simulink model "part3_batterychargingchanged"  (R2022b)
settings: Solver=VariableStepAuto  StartTime=0.0  StopTime=120  RelTol=1e-3
undefined symbols (not defined in the file): High, Low
libraries: fl_lib x6, nesl_utility x6, ee_lib x3, batteryecm_lib x1
settings Model: Creator=mingreico  LastModifiedBy=mingreico

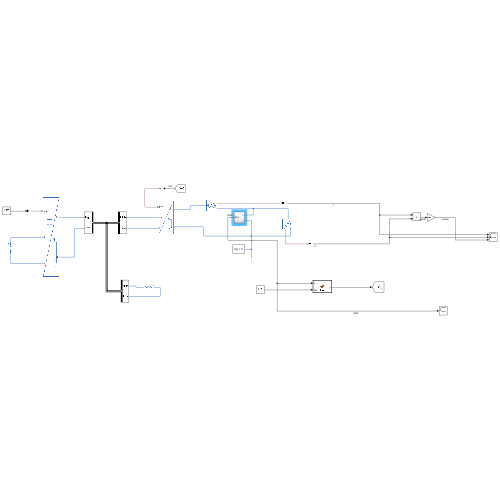
[thumbnail: Simulink's stored preview of the top-level diagram]
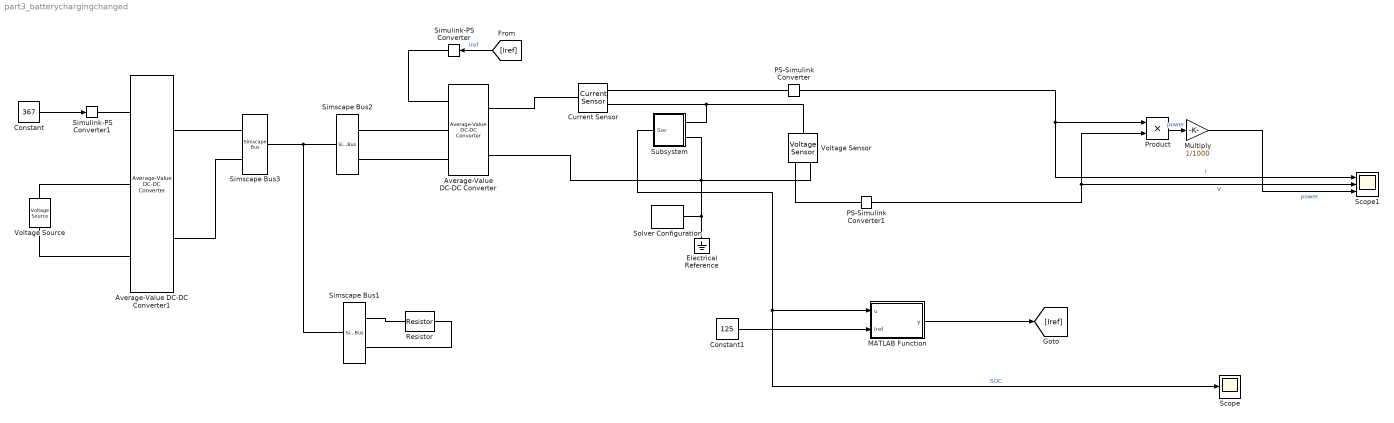
== system part3_batterychargingchanged ==
  Average-Value DC-DC Converter : ee_lib/Semiconductors & Converters/Converters/Average-Value DC-DC Converter  control_option=ee.enum.converters.controlinput.current  converter_type=ee.enum.converters.dcdctype.buckboost  efficiency_option=ee.enum.converters.efficiency.constant  efficiency_fixed=100  i_vec=[0, 2, 5] A  efficiency_vec=[90, 95, 98]
      settings: InternalSimscapePortConfiguration="{\"Bottom\":[],\"Left\":[{\"id\":\"Iref\",\"label\":\"Iref\",\"type\":\"input\"},{\"id\":\"p1\",\"label\":\"1+\",\"type\":\"foundation.electrical.electrical\"},{\"id\":\"n1\",\"label\":\"1-\",\"type\":\"foundation.electrical.electrical\"}],\"Right\":[{\"id\":\"p2\",\"label\":\"2+\",\"type\":\"foundation.electrical.electrical\"},{\"id\":\"n2\",\"label\":\"2-\",\"type\":\"foundation.electrical.electrical\"}],\"Top\":[]}"
  Average-Value DC-DC Converter1 : ee_lib/Semiconductors & Converters/Converters/Average-Value DC-DC Converter  control_option=ee.enum.converters.controlinput.voltage  converter_type=ee.enum.converters.dcdctype.buck  efficiency_option=ee.enum.converters.efficiency.constant  efficiency_fixed=100  i_vec=[0, 2, 5] A  efficiency_vec=[90, 95, 98]
      settings: InternalSimscapePortConfiguration="{\"Bottom\":[],\"Left\":[{\"id\":\"Vref\",\"label\":\"Vref\",\"type\":\"input\"},{\"id\":\"p1\",\"label\":\"1+\",\"type\":\"foundation.electrical.electrical\"},{\"id\":\"n1\",\"label\":\"1-\",\"type\":\"foundation.electrical.electrical\"}],\"Right\":[{\"id\":\"p2\",\"label\":\"2+\",\"type\":\"foundation.electrical.electrical\"},{\"id\":\"n2\",\"label\":\"2-\",\"type\":\"foundation.electrical.electrical\"}],\"Top\":[]}"
  Constant : Constant  Value=367
  Constant1 : Constant  Value=125
  Current Sensor : fl_lib/Electrical/Electrical Sensors/Current Sensor
  Electrical Reference : fl_lib/Electrical/Electrical Elements/Electrical Reference
  MATLAB Function : MATLAB Function  TreatAsAtomicUnit=on
  Multiply : Gain  Gain=1/1000
  PS-Simulink Converter : nesl_utility/PS-Simulink Converter  PhysicalDomain=network_engine_domain  SubClassName=ps_output  LeftPortType=input  RightPortType=output  PseudoPeriodic=off  Frequencies=[]  VectorFormat=inherit  Unit=inherit  AffineConversion=off
  PS-Simulink Converter1 : nesl_utility/PS-Simulink Converter  PhysicalDomain=network_engine_domain  SubClassName=ps_output  LeftPortType=input  RightPortType=output  PseudoPeriodic=off  Frequencies=[]  VectorFormat=inherit  Unit=inherit  AffineConversion=off
  Product : Product
  Resistor : fl_lib/Electrical/Electrical Elements/Resistor  R=1000 Ohm  i_specify=off  i_priority=None  i=0 A  i_nominal_specify=off  i_nominal_unit=A  i_nominal_value=1  v_specify=off  v_priority=None  v=0 V  v_nominal_specify=off  v_nominal_unit=V  v_nominal_value=1
  Scope : Scope
  Scope1 : Scope  NumInputPorts=3
  Simscape Bus1 : SimscapeBus  HierarchyStrings=High;Low
  Simscape Bus2 : SimscapeBus  HierarchyStrings=High;Low
  Simscape Bus3 : SimscapeBus  HierarchyStrings=High;Low
  Simulink-PS Converter : nesl_utility/Simulink-PS Converter  PhysicalDomain=network_engine_domain  SubClassName=ps_input  LeftPortType=input  RightPortType=output  PseudoPeriodic=off  Frequencies=[]  NoiseDistribution=none  NoiseParameters=[]  Unit=1  AffineConversion=off  FilteringAndDerivatives=provide  SimscapeFilterOrder=1  InputFilterTimeConstant=0.001  UdotUserProvided=0
  Simulink-PS Converter1 : nesl_utility/Simulink-PS Converter  PhysicalDomain=network_engine_domain  SubClassName=ps_input  LeftPortType=input  RightPortType=output  PseudoPeriodic=off  Frequencies=[]  NoiseDistribution=none  NoiseParameters=[]  Unit=1  AffineConversion=off  FilteringAndDerivatives=provide  SimscapeFilterOrder=1  InputFilterTimeConstant=0.001  UdotUserProvided=0
  Solver Configuration : nesl_utility/Solver Configuration  PhysicalDomain=network_engine_domain  SubClassName=solver  LeftPortType=input  RightPortType=generic  Tones=[]  Harmonics=[]  SimulateNoise=off  Profile=off  UseLocalSampling=off  EnableSwitchedLinearOptims=on  FrequencyDomain=off  UseCCode=off  RelTol=0.001  AbsTol=0.001  MinStep=1e-09  ToWorkspace=off  RevertToSquareIcSolve=off  NumHomotopyIterations=100  PhasorMode=off  PhasorModeNumHarmonics=1  ConsistencySolver=NEWTON_XTOL_AFTER_FTOL  IndexReductionMethod=DerivativeReplacement  DoDC=off  ResidualTolerance=1e-09  ConsistencyTolSource=GLOBAL  ConsistencyAbsTol=0.001  ConsistencyRelTol=0.001  ConsistencyTolFactor=0.001  UseLocalSolver=off  LocalSolverChoice=NE_BACKWARD_EULER_ADVANCER  ResolveIndetEquations=on  FunctionEvalNumThread=1  LocalSolverSampleTime=0.001  DoFixedCost=off  MaxNonlinIter=3  MaxModeIter=2  ComputeImpulses=off  ImpulseIterations=2  LinearAlgebra=auto  LinearAlgebraNumThread=0  EquationFormulation=NE_TIME_EF  DelaysMemoryBudget=1024  AutomaticFiltering=on  FilteringTimeConstant=0.001  PartitionStorageMethod=AS_NEEDED  PartitionMemoryBudget=1024  PartitionMethod=ROBUST
  Subsystem : Subsystem
  Voltage Sensor : fl_lib/Electrical/Electrical Sensors/Voltage Sensor
  Voltage Source : ee_lib/Sources/Voltage Source  dc_voltage=1000 V  ac_voltage=0 V  ac_shift=0 rad  ac_frequency=60 Hz  noise_mode=ee.enum.sources.noise.Disabled  PSD=0 V^2/Hz  sample_time=1e-3 s  repeatability=ee.enum.sources.repeatability.NotRepeatable  user_seed=0  auto_seed=3890346746  i_specify=off  i_priority=None  i=0 A  i_nominal_specify=off  i_nominal_unit=A  i_nominal_value=1  v_specify=off  v_priority=None  v=0 V  v_nominal_specify=off  v_nominal_unit=V  v_nominal_value=1
  wires:
  PS-Simulink Converter/1 -> Scope1/1, Product/1  "I"
  PS-Simulink Converter1/1 -> Product/2, Scope1/2  "V"
  [Iref] -> Simulink-PS Converter/1  "iref"
  MATLAB Function/1(y) -> [Iref]
  Constant/1 -> Simulink-PS Converter1/1
  Subsystem/1(Soc) -> Scope/1, MATLAB Function/1(u)  "SOC"
  Constant1/1 -> MATLAB Function/2(Iref)
  Product/1 -> Multiply/1  "power"
  Multiply/1 -> Scope1/3  "power"
  connections:
  Current Sensor/RConn2 -- Voltage Sensor/LConn1 -- Subsystem/LConn1
  Current Sensor/RConn1 -- PS-Simulink Converter/LConn1
  Voltage Sensor/RConn1 -- PS-Simulink Converter1/LConn1
  Simulink-PS Converter/RConn1 -- Average-Value DC-DC Converter/LConn1
  Voltage Source/RConn1 -- Average-Value DC-DC Converter1/LConn3
  Simulink-PS Converter1/RConn1 -- Average-Value DC-DC Converter1/LConn1
  Voltage Source/LConn1 -- Average-Value DC-DC Converter1/LConn2
  Simscape Bus3/LConn1 -- Average-Value DC-DC Converter1/RConn1
  Average-Value DC-DC Converter1/RConn2 -- Simscape Bus3/LConn2
  Simscape Bus2/RConn1 -- Simscape Bus1/RConn1 -- Simscape Bus3/RConn1
  Average-Value DC-DC Converter/LConn2 -- Simscape Bus2/LConn1
  Simscape Bus2/LConn2 -- Average-Value DC-DC Converter/LConn3
  Subsystem/LConn2 -- Voltage Sensor/RConn2 -- Average-Value DC-DC Converter/RConn2 -- Solver Configuration/RConn1 -- Electrical Reference/LConn1
  Current Sensor/LConn1 -- Average-Value DC-DC Converter/RConn1
  Resistor/LConn1 -- Simscape Bus1/LConn1
  Resistor/RConn1 -- Simscape Bus1/LConn2

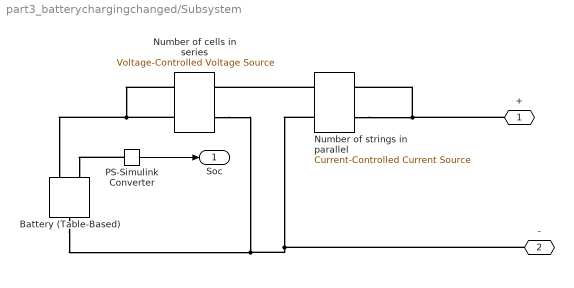
== system part3_batterychargingchanged/Subsystem ==
  Battery (Table-Based) : batteryecm_lib/Battery (Table-Based)  Tag={'toolbox/physmod/battery/shared_library/m/batteryecm_lib_parts';'Battery__Table_Based_/Panasonic/NCR18650PF.xml'}  SOC_vec=[0 0.01 0.02 0.03 0.04 0.05 0.06 0.07 0.08 0.09 0.1 0.11 0.12 0.13 0.14 0.15 0.16 0.17 0.18 0.19 0.2 0.21 0.22 0.23 0.24 0.25 0.26 0.27 0.28 0.29 0.3 0.31 0.32 0.33 0.34 0.35 0.36 0.37 0.38 0.39 0.4 0.41 0.42 0.43 0.44 0.45 0.46 0.47 0.48 0.49 0.5 0.51 0.52 0.53 0.54 0.55 0.56 0.57 0.58 0.59 0.6 0.61 0.62 0.63 0.64 0.65 0.66 0.67 0.68 0.69 0.7 0.71 0.72 0.73 0.74 0.75 0.76 0.77 0.78 0.79 0.8 0.81 0.82 0.83 0.84 0.85 0.86 0.87 0.88 0.89 0.9 0.91 0.92 0.93 0.94 0.95 0.96 0.97 0.98 0.99 1]  T_dependence=simscape.enum.tablebattery.temperature_dependence.yes  prm_dir=simscape.enum.tablebattery.prm_dir.noCurrentDirectionality  T_vec=[-10 0 25 45] degC  V0_mat=[2.80555 2.80555 2.80555 2.80555;2.85959 2.85959 2.85959 2.85959;2.91363 2.91363 2.91363 2.91363;3.00304 3.00304 3.00304 3.00304;3.0606 3.0606 3.0606 3.0606;3.09933 3.09933 3.09933 3.09933;3.12978 3.12978 3.12978 3.12978;3.18381 3.18381 3.18381 3.18381;3.23096 3.23096 3.23096 3.23096;3.26469 3.26469 3.26469 3.26469;3.2911 3.2911 3.2911 3.2911;3.31202 3.31202 3.31202 3.31202;3.33368 3.33368 3.33368 3.33368;3.35023 3.35023 3.35023 3.35023;3.3665 3.3665 3.3665 3.3665;3.38187 3.38187 3.38187 3.38187;3.39652 3.39652 3.39652 3.39652;3.40935 3.40935 3.40935 3.40935;3.42296 3.42296 3.42296 3.42296;3.43602 3.43602 3.43602 3.43602;3.4475 3.4475 3.4475 3.4475;3.45894 3.45894 3.45894 3.45894;3.46943 3.46943 3.46943 3.46943;3.47583 3.47583 3.47583 3.47583;3.48131 3.48131 3.48131 3.48131;3.48929 3.48929 3.48929 3.48929;3.49863 3.49863 3.49863 3.49863;3.50723 3.50723 3.50723 3.50723;3.51419 3.51419 3.51419 3.51419;3.52064 3.52064 3.52064 3.52064;3.52703 3.52703 3.52703 3.52703;3.53288 3.53288 3.53288 3.53288;3.5383 3.5383 3.5383 3.5383;3.54248 3.54248 3.54248 3.54248;3.54635 3.54635 3.54635 3.54635;3.55067 3.55067 3.55067 3.55067;3.55538 3.55538 3.55538 3.55538;3.56162 3.56162 3.56162 3.56162;3.56772 3.56772 3.56772 3.56772;3.57355 3.57355 3.57355 3.57355;3.57907 3.57907 3.57907 3.57907;3.58466 3.58466 3.58466 3.58466;3.59099 3.59099 3.59099 3.59099;3.59795 3.59795 3.59795 3.59795;3.60491 3.60491 3.60491 3.60491;3.61176 3.61176 3.61176 3.61176;3.61856 3.61856 3.61856 3.61856;3.62438 3.62438 3.62438 3.62438;3.62996 3.62996 3.62996 3.62996;3.63625 3.63625 3.63625 3.63625;3.64309 3.64309 3.64309 3.64309;3.64978 3.64978 3.64978 3.64978;3.65633 3.65633 3.65633 3.65633;3.66344 3.66344 3.66344 3.66344;3.67149 3.67149 3.67149 3.67149;3.67995 3.67995 3.67995 3.67995;3.68883 3.68883 3.68883 3.68883;3.69977 3.69977 3.69977 3.69977;3.7106 3.7106 3.7106 3.7106;3.72128 3.72128 3.72128 3.72128;3.72977 3.72977 3.72977 3.72977;3.73862 3.73862 3.73862 3.73862;3.74839 3.74839 3.74839 3.74839;3.75854 3.75854 3.75854 3.75854;3.76808 3.76808 3.76808 3.76808;3.77731 3.77731 3.77731 3.77731;3.78691 3.78691 3.78691 3.78691;3.79724 3.79724 3.79724 3.79724;3.80748 3.80748 3.80748 3.80748;3.817 3.817 3.817 3.817;3.82465 3.82465 3.82465 3.82465;3.83227 3.83227 3.83227 3.83227;3.8402 3.8402 3.8402 3.8402;3.84937 3.84937 3.84937 3.84937;3.85948 3.85948 3.85948 3.85948;3.87001 3.87001 3.87001 3.87001;3.88001 3.88001 3.88001 3.88001;3.88909 3.88909 3.88909 3.88909;3.89708 3.89708 3.89708 3.89708;3.90554 3.90554 3.90554 3.90554;3.91623 3.91623 3.91623 3.91623;3.9276 3.9276 3.9276 3.9276;3.9408 3.9408 3.9408 3.9408;3.95458 3.95458 3.95458 3.95458;3.96671 3.96671 3.96671 3.96671;3.97597 3.97597 3.97597 3.97597;3.98588 3.98588 3.98588 3.98588;3.99921 3.99921 3.99921 3.99921;4.01279 4.01279 4.01279 4.01279;4.02654 4.02654 4.02654 4.02654;4.03959 4.03959 4.03959 4.03959;4.05214 4.05214 4.05214 4.05214;4.06294 4.06294 4.06294 4.06294;4.07257 4.07257 4.07257 4.07257;4.08033 4.08033 4.08033 4.08033;4.08863 4.08863 4.08863 4.08863;4.09953 4.09953 4.09953 4.09953;4.11328 4.11328 4.11328 4.11328;4.13091 4.13091 4.13091 4.13091;4.15201 4.15201 4.15201 4.15201;4.17387 4.17387 4.17387 4.17387] V  V0_vec=[2.80555 2.85959 2.91363 3.00304 3.0606 3.09933 3.12978 3.18381 3.23096 3.26469 3.2911 3.31202 3.33368 3.35023 3.3665 3.38187 3.39652 3.40935 3.42296 3.43602 3.4475 3.45894 3.46943 3.47583 3.48131 3.48929 3.49863 3.50723 3.51419 3.52064 3.52703 3.53288 3.5383 3.54248 3.54635 3.55067 3.55538 3.56162 3.56772 3.57355 3.57907 3.58466 3.59099 3.59795 3.60491 3.61176 3.61856 3.62438 3.62996 3.63625 3.64309 3.64978 3.65633 3.66344 3.67149 3.67995 3.68883 3.69977 3.7106 3.72128 3.72977 3.73862 3.74839 3.75854 3.76808 3.77731 3.78691 3.79724 3.80748 3.817 3.82465 3.83227 3.8402 3.84937 3.85948 3.87001 3.88001 3.88909 3.89708 3.90554 3.91623 3.9276 3.9408 3.95458 3.96671 3.97597 3.98588 3.99921 4.01279 4.02654 4.03959 4.05214 4.06294 4.07257 4.08033 4.08863 4.09953 4.11328 4.13091 4.15201 4.17387] V  V_range=[2.25 Inf] V  R0_mat=[0.75549 0.67245 0.17403 0.112;0.85269 0.75703 0.14702 0.03414;0.81792 0.71964 0.12022 0.00255;0.78315 0.68225 0.10415 2e-05;0.74837 0.64486 0.08835 2e-05;0.7136 0.60747 0.07462 2e-05;0.67883 0.57008 0.06392 2e-05;0.64406 0.53269 0.06243 0.01154;0.60929 0.49529 0.06276 0.02196;0.57452 0.4579 0.06157 0.02895;0.53975 0.42051 0.06015 0.03291;0.50498 0.38312 0.0587 0.03446;0.47021 0.34573 0.05791 0.03749;0.43544 0.30834 0.05742 0.03912;0.40067 0.27163 0.05726 0.04077;0.3659 0.2399 0.05695 0.04312;0.33113 0.21598 0.05669 0.04519;0.29855 0.19556 0.0563 0.04597;0.27187 0.18199 0.05643 0.04689;0.25149 0.16998 0.05637 0.04778;0.23672 0.15947 0.05613 0.04881;0.22094 0.15288 0.05627 0.04983;0.21055 0.14641 0.0562 0.05042;0.19955 0.13998 0.0555 0.04905;0.19137 0.13379 0.05463 0.04734;0.18464 0.13036 0.05424 0.0468;0.17901 0.12743 0.05396 0.04733;0.17336 0.12471 0.05353 0.04759;0.16963 0.12142 0.05325 0.04697;0.16579 0.11998 0.053 0.04616;0.16242 0.11856 0.05273 0.04563;0.15887 0.11696 0.05239 0.04515;0.15558 0.1153 0.05185 0.04523;0.15182 0.11319 0.05104 0.04515;0.14868 0.11098 0.05016 0.04495;0.14619 0.10898 0.0496 0.04427;0.1438 0.10712 0.04917 0.0435;0.14196 0.10583 0.049 0.0433;0.14006 0.10467 0.04873 0.04342;0.13885 0.1036 0.04841 0.04343;0.13751 0.10241 0.04805 0.04333;0.13605 0.10125 0.04775 0.04289;0.13479 0.10081 0.04765 0.04219;0.13386 0.10079 0.04766 0.04172;0.13314 0.10076 0.04767 0.04125;0.13237 0.10071 0.04767 0.04141;0.13163 0.10106 0.04767 0.04164;0.13057 0.10103 0.04746 0.04127;0.12942 0.10092 0.04718 0.04039;0.12835 0.0993 0.04683 0.03977;0.12742 0.09756 0.04661 0.03935;0.12651 0.09576 0.04638 0.03877;0.12576 0.09551 0.04611 0.03814;0.12522 0.09549 0.04546 0.03775;0.12534 0.0958 0.04498 0.03789;0.12567 0.09566 0.0446 0.03806;0.12544 0.09568 0.04436 0.03754;0.12563 0.09645 0.0447 0.03778;0.12579 0.09742 0.0452 0.03809;0.12561 0.09838 0.04568 0.03858;0.12463 0.09848 0.04568 0.03827;0.12444 0.09858 0.04565 0.03791;0.12488 0.09902 0.04553 0.03774;0.12541 0.0989 0.04551 0.03771;0.12553 0.09832 0.04545 0.0378;0.12554 0.09763 0.04533 0.03827;0.12569 0.09779 0.04532 0.03888;0.12679 0.09822 0.0455 0.03964;0.12813 0.09884 0.04565 0.03957;0.12921 0.09949 0.04568 0.03924;0.12875 0.09944 0.04547 0.03856;0.12761 0.09947 0.04525 0.03793;0.12678 0.09962 0.04509 0.0374;0.12741 0.10014 0.04486 0.03728;0.12819 0.10071 0.04471 0.03749;0.12866 0.10143 0.04473 0.03825;0.12934 0.10218 0.04488 0.0389;0.13071 0.10266 0.04509 0.03921;0.13167 0.10268 0.04508 0.03827;0.13235 0.10275 0.04519 0.03748;0.13367 0.10365 0.04567 0.03751;0.13524 0.10475 0.0459 0.03791;0.1378 0.10652 0.04653 0.03898;0.14098 0.10898 0.04736 0.0402;0.14355 0.11127 0.04774 0.04039;0.14492 0.11249 0.04743 0.03953;0.1465 0.11343 0.04723 0.03861;0.14934 0.11546 0.04771 0.03891;0.15255 0.11759 0.04823 0.0391;0.15585 0.12007 0.04878 0.03936;0.15888 0.12238 0.04933 0.0398;0.16256 0.12454 0.04973 0.04018;0.16629 0.12609 0.0497 0.03988;0.16958 0.1272 0.04945 0.03914;0.1737 0.12779 0.0488 0.0377;0.17938 0.12952 0.04782 0.03647;0.18591 0.1322 0.04663 0.0362;0.19342 0.13509 0.04586 0.03591;0.20235 0.13879 0.04557 0.03672;0.20886 0.14194 0.04146 0.03487;0.20094 0.13122 0.03511 0.0299] Ohm  R0_vec=[0.17403 0.14702 0.12022 0.10415 0.08835 0.07462 0.06392 0.06243 0.06276 0.06157 0.06015 0.0587 0.05791 0.05742 0.05726 0.05695 0.05669 0.0563 0.05643 0.05637 0.05613 0.05627 0.0562 0.0555 0.05463 0.05424 0.05396 0.05353 0.05325 0.053 0.05273 0.05239 0.05185 0.05104 0.05016 0.0496 0.04917 0.049 0.04873 0.04841 0.04805 0.04775 0.04765 0.04766 0.04767 0.04767 0.04767 0.04746 0.04718 0.04683 0.04661 0.04638 0.04611 0.04546 0.04498 0.0446 0.04436 0.0447 0.0452 0.04568 0.04568 0.04565 0.04553 0.04551 0.04545 0.04533 0.04532 0.0455 0.04565 0.04568 0.04547 0.04525 0.04509 0.04486 0.04471 0.04473 0.04488 0.04509 0.04508 0.04519 0.04567 0.0459 0.04653 0.04736 0.04774 0.04743 0.04723 0.04771 0.04823 0.04878 0.04933 0.04973 0.0497 0.04945 0.0488 0.04782 0.04663 0.04586 0.04557 0.04146 0.03511] Ohm  R0_dis_mat=[.0117, .0085, .009; .011, .0085, .009; .0114, .0087, .0092; .0107, .0082, .0088; .0107, .0083, .0091; .0113, .0085, .0089; .0116, .0085, .0089] % Parameter not set Ohm  R0_dis_vec=[.0085, .0085, .0087, .0082, .0083, .0085, .0085] % Parameter not set Ohm  R0_ch_mat=[.0117, .0085, .009; .011, .0085, .009; .0114, .0087, .0092; .0107, .0082, .0088; .0107, .0083, .0091; .0113, .0085, .0089; .0116, .0085, .0089] % Parameter not set Ohm  R0_ch_vec=[.0085, .0085, .0087, .0082, .0083, .0085, .0085] % Parameter not set Ohm  AH=1.9 Ah  prm_leak=simscape.enum.tablebattery.prm_leak.disabled  Rleak_vec=[8000, 7000, 6000] % Parameter not set Ohm  Rleak=7e3 % Parameter not set Ohm  extrapolation_option=simscape.enum.extrapolation.nearest  SOC_port=simscape.enum.tablebattery.enable.yes  prm_dyn=simscape.enum.tablebattery.prm_dyn.off  R1_mat=[.0109, .0029, .0013; .0069, .0024, .0012; .0047, .0026, .0013; .0034, .0016, .001; .0033, .0023, .0014; .0033, .0018, .0011; .0028, .0017, .0011] % Parameter not set Ohm  R1_vec=[.0029, .0024, .0026, .0016, .0023, .0018, .0017] % Parameter not set Ohm  tau1_mat=[20, 36, 39; 31, 45, 39; 109, 105, 61; 36, 29, 26; 59, 77, 67; 40, 33, 29; 25, 39, 33] % Parameter not set s  tau1_vec=[36, 45, 105, 29, 77, 33, 39] % Parameter not set s  R2_mat=[.0109, .0029, .0013; .0069, .0024, .0012; .0047, .0026, .0013; .0034, .0016, .001; .0033, .0023, .0014; .0033, .0018, .0011; .0028, .0017, .0011] % Parameter not set Ohm  R2_vec=[.0029, .0024, .0026, .0016, .0023, .0018, .0017] % Parameter not set Ohm  tau2_mat=[20, 36, 39; 31, 45, 39; 109, 105, 61; 36, 29, 26; 59, 77, 67; 40, 33, 29; 25, 39, 33] % Parameter not set s  tau2_vec=[36, 45, 105, 29, 77, 33, 39] % Parameter not set s  R3_mat=[.0109, .0029, .0013; .0069, .0024, .0012; .0047, .0026, .0013; .0034, .0016, .001; .0033, .0023, .0014; .0033, .0018, .0011; .0028, .0017, .0011] % Parameter not set Ohm  R3_vec=[.0029, .0024, .0026, .0016, .0023, .0018, .0017] % Parameter not set Ohm  tau3_mat=[20, 36, 39; 31, 45, 39; 109, 105, 61; 36, 29, 26; 59, 77, 67; 40, 33, 29; 25, 39, 33] % Parameter not set s  tau3_vec=[36, 45, 105, 29, 77, 33, 39] % Parameter not set s  R4_mat=[.0109, .0029, .0013; .0069, .0024, .0012; .0047, .0026, .0013; .0034, .0016, .001; .0033, .0023, .0014; .0033, .0018, .0011; .0028, .0017, .0011] % Parameter not set Ohm  R4_vec=[.0029, .0024, .0026, .0016, .0023, .0018, .0017] % Parameter not set Ohm  tau4_mat=[20, 36, 39; 31, 45, 39; 109, 105, 61; 36, 29, 26; 59, 77, 67; 40, 33, 29; 25, 39, 33] % Parameter not set s  tau4_vec=[36, 45, 105, 29, 77, 33, 39] % Parameter not set s  R5_mat=[.0109, .0029, .0013; .0069, .0024, .0012; .0047, .0026, .0013; .0034, .0016, .001; .0033, .0023, .0014; .0033, .0018, .0011; .0028, .0017, .0011] % Parameter not set Ohm  R5_vec=[.0029, .0024, .0026, .0016, .0023, .0018, .0017] % Parameter not set Ohm  tau5_mat=[20, 36, 39; 31, 45, 39; 109, 105, 61; 36, 29, 26; 59, 77, 67; 40, 33, 29; 25, 39, 33] % Parameter not set s  tau5_vec=[36, 45, 105, 29, 77, 33, 39] % Parameter not set s  prm_fade=simscape.enum.tablebattery.prm_fade.tableN  N0=100 % Parameter not set  dV0=0 % Parameter not set  dR0=0 % Parameter not set  dAH=0 % Parameter not set  dRleak=0 % Parameter not set  dR1=0 % Parameter not set  dR2=0 % Parameter not set  dR3=0 % Parameter not set  dR4=0 % Parameter not set  dR5=0 % Parameter not set  N0vec=[1 7 13 19 25 31 37 43 49 55 61 67 73 79 85 91 97 103 109 115 121 127 133 139 145 151 157 163 169 175 181 187 193 199 205 211 217 223 229 235 241 247 253 259 265 271 277 283 289 295 301 307 313 319 325 331 337 343 349 355 361 367 373 379 385 391 397 403 409 415 421 427 433 439 445 451 457 463 469 475 481 487 493 499]  Tfadevec=[298.15, 323.15] % Parameter not set K  dV0vec=[0 -0.2132 -0.4265 -0.6357 -0.8415 -1.0444 -1.2163 -1.3883 -1.52 -1.6273 -1.7347 -1.8294 -1.9144 -1.9994 -2.0744 -2.1392 -2.204 -2.2607 -2.3098 -2.3589 -2.408 -2.4643 -2.5252 -2.5861 -2.647 -2.7238 -2.8051 -2.8864 -2.9759 -3.0704 -3.1649 -3.261 -3.3591 -3.4573 -3.5079 -3.5566 -3.6065 -3.6564 -3.7063 -3.7562 -3.8061 -3.8559 -3.9166 -3.9805 -4.0444 -4.1083 -4.1723 -4.2352 -4.2979 -4.3605 -4.4214 -4.4739 -4.5206 -4.5597 -4.5988 -4.6379 -4.6769 -4.716 -4.7547 -4.7957 -4.8368 -4.8778 -4.9188 -4.9598 -5.0123 -5.066 -5.1196 -5.1598 -5.1853 -5.2109 -5.2365 -5.2631 -5.2922 -5.3213 -5.3503 -5.3816 -5.4144 -5.4471 -5.4798 -5.5126 -5.5453 -5.578 -5.6097 -5.641]  dR0vec=[0 0 0 0 0 0 0 0 0 0 0 0 0 0 0 0 0 0 0 0 0 0 0 0 0 0 0 0 0 0 0 0 0 0 0 0 0 0 0 0 0 0 0 0 0 0 0 0 0 0 0 0 0 0 0 0 0 0 0 0 0 0 0 0 0 0 0 0 0 0 0 0 0 0 0 0 0 0 0 0 0 0 0 0] % Parameter assumed  dAHvec=[0 -0.407 -0.814 -1.221 -1.629 -2.036 -2.443 -2.85 -3.207 -3.533 -3.859 -4.185 -4.51 -4.836 -5.162 -5.488 -5.813 -6.105 -6.369 -6.633 -6.897 -7.161 -7.425 -7.689 -7.953 -8.255 -8.569 -8.883 -9.197 -9.511 -9.826 -10.14 -10.454 -10.768 -10.93 -11.081 -11.233 -11.384 -11.536 -11.687 -11.838 -11.99 -12.176 -12.372 -12.569 -12.765 -12.962 -13.158 -13.354 -13.551 -13.741 -13.906 -14.07 -14.235 -14.399 -14.564 -14.728 -14.893 -15.06 -15.244 -15.429 -15.614 -15.799 -15.983 -16.168 -16.353 -16.538 -16.676 -16.764 -16.852 -16.94 -17.028 -17.116 -17.204 -17.292 -17.387 -17.486 -17.585 -17.684 -17.783 -17.883 -17.982 -18.081 -18.18]  dRleakvec=[0, 0, 0] % Parameter not set  dR1vec=[0, 0, 0] % Parameter not set  dR2vec=[0, 0, 0] % Parameter not set  dR3vec=[0, 0, 0] % Parameter not set  dR4vec=[0, 0, 0] % Parameter not set  dR5vec=[0, 0, 0] % Parameter not set  dV0mat=[0, 0; 0, 0; 0, 0] % Parameter not set  dR0mat=[0, 0; 0, 0; 0, 0] % Parameter not set  dAHmat=[0, 0; 0, 0; 0, 0] % Parameter not set  dRleakmat=[0, 0; 0, 0; 0, 0] % Parameter not set  dR1mat=[0, 0; 0, 0; 0, 0] % Parameter not set  dR2mat=[0, 0; 0, 0; 0, 0] % Parameter not set  dR3mat=[0, 0; 0, 0; 0, 0] % Parameter not set  dR4mat=[0, 0; 0, 0; 0, 0] % Parameter not set  dR5mat=[0, 0; 0, 0; 0, 0] % Parameter not set  prm_age_modeling=simscape.enum.tablebattery.prm_age_modeling.equation  storage_dt_age_vec=[0] % Parameter not set d  storage_T_age_vec=[273] % Parameter not set K  prm_age_OCV=simscape.enum.tablebattery.prm_age_OCV.OCV  OCV_age=0.9 % Parameter not set  SOC_age=0.6 % Parameter not set  prm_age_resistance=simscape.enum.tablebattery.prm_age.disabled  OCV_scaling_age_resistance=2.2134e6 % Parameter not set  OCV_offset_age_resistance=1.632e6 % Parameter not set  temp_exp_age_resistance=0.515833569 % Parameter not set V  t_exp_age_resistance=0.75 % Parameter not set  T_age_vec_resistance=[273.15, 298.15, 323.15] % Parameter not set K  dt_age_vec_resistance=[90, 180, 270, 360] % Parameter not set d  dR0_age_vec=[0, 0, 0] % Parameter not set  t_meas_dR0_age=100 % Parameter not set d  dR0_age_mat=[0, 0, 0; 0, 0, 0; 0, 0, 0; 0, 0, 0] % Parameter not set  prm_age_capacity=simscape.enum.tablebattery.prm_age.disabled  OCV_scaling_age_capacity=1.5097e07 % Parameter not set  OCV_offset_age_capacity=8.3625e06 % Parameter not set  temp_exp_age_capacity=0.6011 % Parameter not set V  t_exp_age_capacity=0.75 % Parameter not set  T_age_vec_capacity=[273.15, 298.15, 323.15] % Parameter not set K  dt_age_vec_capacity=[90, 180, 270, 360] % Parameter not set d  dAH_age_vec=[0, 0, 0] % Parameter not set  t_meas_dAH_age=100 % Parameter not set d  dAH_age_mat=[0, 0, 0; 0, 0, 0; 0, 0, 0; 0, 0, 0] % Parameter not set  thermal_port=simscape.enum.thermaleffects.omit  temperature=298.15 % Parameter not set K  thermal_mass=43.2 % Parameter assumed J/K  i_specify=off  i_priority=None  i=0 A  i_nominal_specify=off  i_nominal_unit=A  i_nominal_value=1  v_specify=off  v_priority=None  v=0 V  v_nominal_specify=off  v_nominal_unit=V  v_nominal_value=1  stateOfCharge_specify=on  stateOfCharge_priority=High  stateOfCharge=0.2  stateOfCharge_nominal_specify=off  stateOfCharge_nominal_unit=1  stateOfCharge_nominal_value=1  num_cycles_specify=off  num_cycles_priority=High  num_cycles=0  num_cycles_nominal_specify=off  num_cycles_nominal_unit=1  num_cycles_nominal_value=1  cell_temperature_specify=off  cell_temperature_priority=High  cell_temperature=298.15 K  cell_temperature_nominal_specify=off  cell_temperature_nominal_unit=K  cell_temperature_nominal_value=1
      settings: AttributesFormatString=Panasonic:NCR18650PF  InternalSimscapePortConfiguration="{\"Bottom\":[],\"Left\":[{\"id\":\"p\",\"label\":\"+\",\"type\":\"foundation.electrical.electrical\"},{\"id\":\"soc\",\"label\":\"SOC\",\"type\":\"output\"}],\"Right\":[{\"id\":\"n\",\"label\":\"-\",\"type\":\"foundation.electrical.electrical\"}],\"Top\":[]}"
  Number of cells in series : fl_lib/Electrical/Electrical Sources/Voltage-Controlled Voltage Source  K=-100  v1_specify=off  v1_priority=None  v1=0 V  v1_nominal_specify=off  v1_nominal_unit=V  v1_nominal_value=1  v2_specify=off  v2_priority=None  v2=0 V  v2_nominal_specify=off  v2_nominal_unit=V  v2_nominal_value=1
      settings: InternalSimscapePortConfiguration="{\"Bottom\":[],\"Left\":[{\"id\":\"p1\",\"label\":\"+\",\"type\":\"foundation.electrical.electrical\"},{\"id\":\"p2\",\"label\":\"+\",\"type\":\"foundation.electrical.electrical\"}],\"Right\":[{\"id\":\"n1\",\"label\":\"-\",\"type\":\"foundation.electrical.electrical\"},{\"id\":\"n2\",\"label\":\"-\",\"type\":\"foundation.electrical.electrical\"}],\"Top\":[]}"
  Number of strings in parallel : fl_lib/Electrical/Electrical Sources/Current-Controlled Current Source  K=-1  i1_specify=off  i1_priority=None  i1=0 A  i1_nominal_specify=off  i1_nominal_unit=A  i1_nominal_value=1  i2_specify=off  i2_priority=None  i2=0 A  i2_nominal_specify=off  i2_nominal_unit=A  i2_nominal_value=1
      settings: InternalSimscapePortConfiguration="{\"Bottom\":[],\"Left\":[{\"id\":\"p1\",\"label\":\"+\",\"type\":\"foundation.electrical.electrical\"},{\"id\":\"head\",\"label\":\"\",\"type\":\"foundation.electrical.electrical\"}],\"Right\":[{\"id\":\"n1\",\"label\":\"-\",\"type\":\"foundation.electrical.electrical\"},{\"id\":\"tail\",\"label\":\"\",\"type\":\"foundation.electrical.electrical\"}],\"Top\":[]}"
  PS-Simulink Converter : nesl_utility/PS-Simulink Converter  PhysicalDomain=network_engine_domain  SubClassName=ps_output  LeftPortType=input  RightPortType=output  PseudoPeriodic=off  Frequencies=[]  VectorFormat=inherit  Unit=inherit  AffineConversion=off
  + : PMIOPort  Side=Left
  - : PMIOPort  Port=2  Side=Left
  Soc : Outport
  wires:
  PS-Simulink Converter/1 -> Soc/1
  connections:
  Number of cells in series/RConn1 -- Number of cells in series/RConn2 -- Battery (Table-Based)/LConn1
  Battery (Table-Based)/RConn1 -- -/RConn1 -- Number of strings in parallel/LConn2 -- Number of cells in series/LConn1
  Number of strings in parallel/LConn1 -- Number of cells in series/LConn2
  Number of strings in parallel/RConn2 -- +/RConn1 -- Number of strings in parallel/RConn1
  PS-Simulink Converter/LConn1 -- Battery (Table-Based)/LConn2

== matlab function part3_batterychargingchanged/MATLAB Function ==
  data: u input; y output; Iref input
function y = fcn(u,Iref)
    if u>=1
        y=0;
    elseif u>=0.8
        y=Iref*0.6;
    else
        y=Iref;
    end
end
